simulink model "ex3"  (R2020a)
settings: Solver=VariableStepAuto  StartTime=0.0  StopTime=10.0  RelTol=1e-3

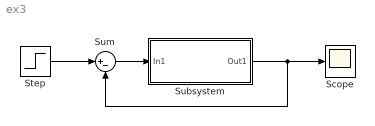
== system ex3 ==
  Scope : Scope
  Step : Step  SampleTime=0
  Subsystem : Subsystem  mask{a=4, b=36}
      mask prompts: a "a="; b "b="
      mask Callback a:
      | if str2num(get_param(gcb,'a'))<0
      |     error('Introduceti o valoare pozitiva pentru a')
      | end
      mask Callback b:
      | if str2num(get_param(gcb,'b'))<0
      |     error('Introduceti o valoare pozitiva pentru b')
      | end
  Sum : Sum  Inputs=|+-
  wires:
  Subsystem/1(Out1) -> Sum/2, Scope/1
  Step/1 -> Sum/1
  Sum/1 -> Subsystem/1(In1)

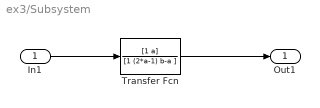
== system ex3/Subsystem ==
  In1 : Inport
  Transfer Fcn : TransferFcn  Numerator=[1 a]  Denominator=[1 (2*a-1) b-a ]
  Out1 : Outport
  wires:
  In1/1 -> Transfer Fcn/1
  Transfer Fcn/1 -> Out1/1
